simulink model "untitled"  (R2018a)
settings: Solver=FixedStepDiscrete  StartTime=0.0  StopTime=inf  RelTol=1e-3  EnableMultiTasking=on
libraries: audiosources x1
settings Model: Creator=gianc  LastModifiedBy=gianc

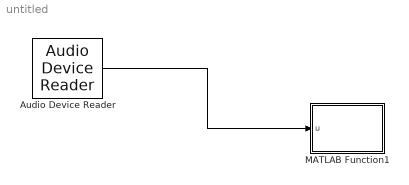
== system untitled ==
  Audio Device Reader : audiosources/Audio Device Reader  Driver=DirectSound  Device=Microfono (2- USB PnP Sound Device)  SampleRate=44100  NumChannels=1  SamplesPerFrame=1024  BitDepth=16-bit integer  NumBuffers=10  DefaultInputChannelMapping=on  InputChannelMapping=1:2  OutputNumOverrunSamples=off  OutputDataType=double  DriverIdx=1  DeviceWarnFlag=''
      settings: SourceProductName=Audio System Toolbox  SourceProductBaseCode=AU
  MATLAB Function1 : MATLAB Function  TreatAsAtomicUnit=on
  wires:
  Audio Device Reader/1 -> MATLAB Function1/1(u)

== matlab function untitled/MATLAB Function1 ==
  data: u input
function fcn(u)
persistent t
if isempty(t)
    t=ones(1024,1);
else
    t(1)=t(1024)+1;
end

for i=1:1023
    t(i+1)=t(i)+1;
end

hold on
plot(t,u,'g');

end
